simulink model "semana1"  (R2019b)
settings: Solver=ode45  StartTime=0.0  StopTime=2500  MaxStep=0.1  RelTol=1e-3
undefined symbols (not defined in the file): A, B, C, D, xini
libraries: cstblocks x1
settings Model: Creator=B13  LastModifiedBy=B13

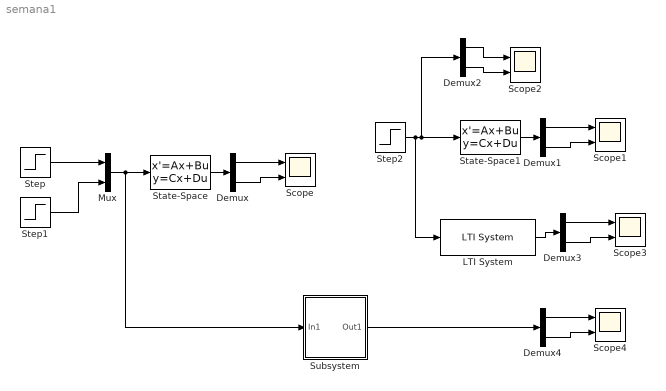
== system semana1 ==
  Demux{,1..4} (5 alike) : Demux  Outputs=2
  LTI System : cstblocks/LTI System  sys=sys  IC=xini
  Mux : Mux  Inputs=2
  Scope{,1..4} (5 alike) : Scope  NumInputPorts=2
  State-Space : StateSpace  A=A  B=B  C=C  D=D  InitialCondition=0
  State-Space1 : StateSpace  A=A  B=B  C=C  D=D  InitialCondition=xini
  Step : Step  Before=1  SampleTime=0
  Step1 : Step  Time=0  After=0  SampleTime=0
  Step2 : Step  Time=[0;0]  Before=[0;0]  After=[1;0]  SampleTime=0
  Subsystem : Subsystem
  wires:
  Mux/1 -> Subsystem/1(In1), State-Space/1
  Step/1 -> Mux/1
  Step1/1 -> Mux/2
  State-Space/1 -> Demux/1
  Demux/1 -> Scope/1
  Demux/2 -> Scope/2
  Demux1/1 -> Scope1/1
  Step2/1 -> LTI System/1, Demux2/1, State-Space1/1
  Demux1/2 -> Scope1/2
  State-Space1/1 -> Demux1/1
  Demux2/2 -> Scope2/2
  Demux2/1 -> Scope2/1
  Demux3/1 -> Scope3/1
  LTI System/1 -> Demux3/1
  Demux3/2 -> Scope3/2
  Demux4/2 -> Scope4/2
  Demux4/1 -> Scope4/1
  Subsystem/1(Out1) -> Demux4/1

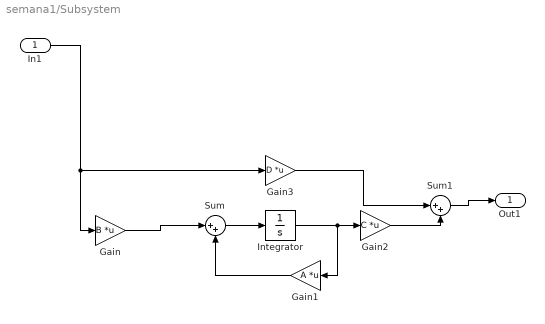
== system semana1/Subsystem ==
  In1 : Inport
  Gain : Gain  Gain=B  Multiplication=Matrix(K*u)
  Gain1 : Gain  Gain=A  Multiplication=Matrix(K*u)
  Gain2 : Gain  Gain=C  Multiplication=Matrix(K*u)
  Gain3 : Gain  Gain=D  Multiplication=Matrix(K*u)
  Integrator : Integrator  InitialCondition=xini
  Sum : Sum  Inputs=|++
  Sum1 : Sum  Inputs=|++
  Out1 : Outport
  wires:
  Sum/1 -> Integrator/1
  Integrator/1 -> Gain1/1, Gain2/1
  Gain/1 -> Sum/1
  Gain3/1 -> Sum1/1
  In1/1 -> Gain/1, Gain3/1
  Gain2/1 -> Sum1/2
  Gain1/1 -> Sum/2
  Sum1/1 -> Out1/1
